simulink subsystem "RelayBoard"  (R2022a)
settings: Solver=VariableStepAuto  StartTime=0.0  StopTime=10.0  RelTol=1e-3
libraries: ee_lib x8, nesl_utility x2
settings Model: Creator=mateu  LastModifiedBy=mateu

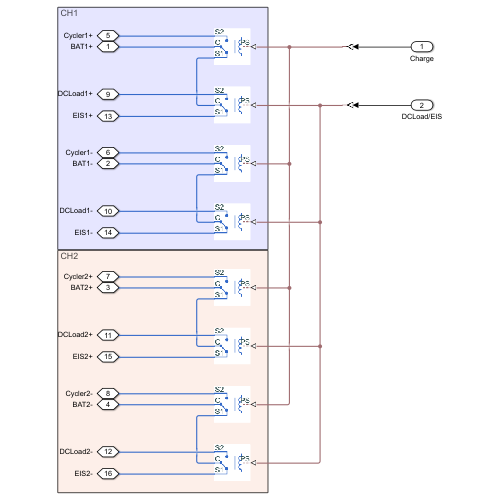
[thumbnail: Simulink's stored preview of the top-level diagram]
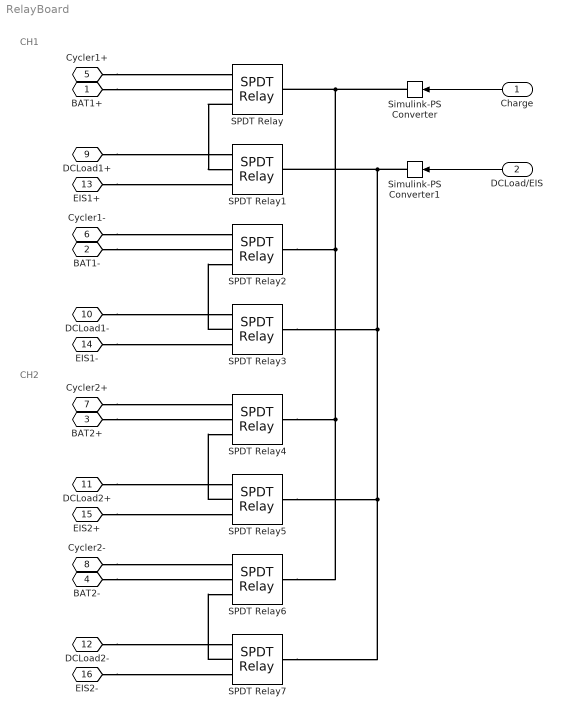
== system RelayBoard ==
  note: CH1
  note: CH2
  Charge : Inport
  DCLoad/EIS : Inport  Port=2
  SPDT Relay{,1..7} (8 alike) : ee_lib/Switches & Breakers/Relays/SPDT Relay  block_choices=ee.enum.controlport.ps  R_closed=0.01 Ohm  G_open=1e-8 1/Ohm  Threshold=0  exposemeasurement=ee.enum.exposemeasurement.hidden  port_locations_spdt=ee.enum.relays.port_locations_spdt.standard  V_rated=5 V  V_energize=75  V_deenergize=25  l_winding=0.08 H  r_winding=12.5 Ohm  g_winding=1e-9 1/Ohm  T_brk_C_S1=0 s  T_mak_C_S1=0 s  T_brk_C_S2=0 s  T_mak_C_S2=0 s  enable_faults=ee.enum.relays.enable.no  fault_action=ee.enum.relays.faultaction.none  fault_types=ee.enum.relays.faultTypes.winding  fault_condition_ps=ee.enum.relays.faultConditionSPDTps.cs1stuck  r_deg_closed_s1=1e-9 Ohm  r_deg_closed_s2=1e-9 Ohm  winding_tau_fault=1e-3 s  tau_fault=1e-3 s  enable_temporal_fault=ee.enum.relays.enable.no  t_fault_stick=1 s  t_fault_ComOpen=1 s  t_fault=1 s  enable_behavioral_fault=ee.enum.relays.enable.no  winding_max_permissible_voltage=inf V  n_fail_on_voltage=1  winding_max_permissible_current=inf A  max_permissible_current=inf A  t_fail_on_current=1 s
      settings: SourceProductBaseCode=PS  InternalSimscapePortConfiguration="{\"Bottom\":[],\"Left\":[{\"id\":\"PS\",\"label\":\"PS\",\"type\":\"input\"}],\"Right\":[{\"id\":\"S2\",\"label\":\"S2\",\"type\":\"foundation.electrical.electrical\"},{\"id\":\"COM\",\"label\":\"C\",\"type\":\"foundation.electrical.electrical\"},{\"id\":\"S1\",\"label\":\"S1\",\"type\":\"foundation.electrical.electrical\"}],\"Top\":[]}"
  Simulink-PS Converter : nesl_utility/Simulink-PS Converter  PhysicalDomain=network_engine_domain  SubClassName=ps_input  LeftPortType=input  RightPortType=output  PseudoPeriodic=off  Frequencies=[]  NoiseDistribution=none  NoiseParameters=[]  Unit=1  AffineConversion=off  FilteringAndDerivatives=provide  SimscapeFilterOrder=1  InputFilterTimeConstant=0.001  UdotUserProvided=0
      settings: SourceProductBaseCode=SS,PW,VE
  Simulink-PS Converter1 : nesl_utility/Simulink-PS Converter  PhysicalDomain=network_engine_domain  SubClassName=ps_input  LeftPortType=input  RightPortType=output  PseudoPeriodic=off  Frequencies=[]  NoiseDistribution=none  NoiseParameters=[]  Unit=1  AffineConversion=off  FilteringAndDerivatives=provide  SimscapeFilterOrder=1  InputFilterTimeConstant=0.001  UdotUserProvided=0
      settings: SourceProductBaseCode=SS,PW,VE
  BAT1+ : PMIOPort  Side=Left
  BAT1- : PMIOPort  Port=2  Side=Left
  BAT2+ : PMIOPort  Port=3  Side=Left
  BAT2- : PMIOPort  Port=4  Side=Left
  Cycler1+ : PMIOPort  Port=5  Side=Left
  Cycler1- : PMIOPort  Port=6  Side=Left
  Cycler2+ : PMIOPort  Port=7  Side=Left
  Cycler2- : PMIOPort  Port=8  Side=Left
  DCLoad1+ : PMIOPort  Port=9  Side=Right
  DCLoad1- : PMIOPort  Port=10  Side=Right
  DCLoad2+ : PMIOPort  Port=11  Side=Right
  DCLoad2- : PMIOPort  Port=12  Side=Right
  EIS1+ : PMIOPort  Port=13  Side=Right
  EIS1- : PMIOPort  Port=14  Side=Right
  EIS2+ : PMIOPort  Port=15  Side=Right
  EIS2- : PMIOPort  Port=16  Side=Right
  wires:
  Charge/1 -> Simulink-PS Converter/1
  DCLoad/EIS/1 -> Simulink-PS Converter1/1
  connections:
  SPDT Relay6/LConn1 -- SPDT Relay4/LConn1 -- SPDT Relay2/LConn1 -- Simulink-PS Converter/RConn1 -- SPDT Relay/LConn1
  SPDT Relay7/LConn1 -- SPDT Relay5/LConn1 -- SPDT Relay3/LConn1 -- Simulink-PS Converter1/RConn1 -- SPDT Relay1/LConn1
  BAT1+/RConn1 -- SPDT Relay/RConn2
  BAT2-/RConn1 -- SPDT Relay6/RConn2
  DCLoad2+/RConn1 -- SPDT Relay5/RConn1
  EIS2-/RConn1 -- SPDT Relay7/RConn3
  DCLoad1+/RConn1 -- SPDT Relay1/RConn1
  BAT1-/RConn1 -- SPDT Relay2/RConn2
  SPDT Relay5/RConn2 -- SPDT Relay4/RConn3
  EIS1-/RConn1 -- SPDT Relay3/RConn3
  DCLoad1-/RConn1 -- SPDT Relay3/RConn1
  EIS2+/RConn1 -- SPDT Relay5/RConn3
  Cycler1-/RConn1 -- SPDT Relay2/RConn1
  Cycler2+/RConn1 -- SPDT Relay4/RConn1
  Cycler2-/RConn1 -- SPDT Relay6/RConn1
  BAT2+/RConn1 -- SPDT Relay4/RConn2
  SPDT Relay/RConn3 -- SPDT Relay1/RConn2
  DCLoad2-/RConn1 -- SPDT Relay7/RConn1
  EIS1+/RConn1 -- SPDT Relay1/RConn3
  SPDT Relay7/RConn2 -- SPDT Relay6/RConn3
  Cycler1+/RConn1 -- SPDT Relay/RConn1
  SPDT Relay3/RConn2 -- SPDT Relay2/RConn3
